simulink model "Proj2_INLC2"  (R2019b)
settings: Solver=VariableStepAuto  StartTime=0.0  StopTime=10.0  RelTol=1e-3
values from neighbouring files (symbols this model uses):
  a_phi_des = pi/2    (= 1.57079632679)    [project2_code.m]
  alpha_NL = 25    [project2_code.m]
  b_phi_des = [pi/2, pi/4]    [project2_code.m]
  beta_NL = 1    [project2_code.m]
  f_phi_des = 0.2    [project2_code.m]
  g = 9.8    [project2_code.m]
  Gamma_NL = eye(5)*1e-9    [project2_code.m]
  phi_des_bar = [pi/8, pi/4]    [project2_code.m]
  phi_dot_IC = [0; 0]    [project2_code.m]
  phi_dotdot_IC = [0; 0]    [project2_code.m]
  THD_IC = new_theta    [project2_code.m]
  theta = [theta1, theta2, theta3, theta4, theta5]    [project2_code.m]
settings Model: Creator=kaush  LastModifiedBy=kaush
settings DebuggingCC: SFMachineParentedDataDiag=error

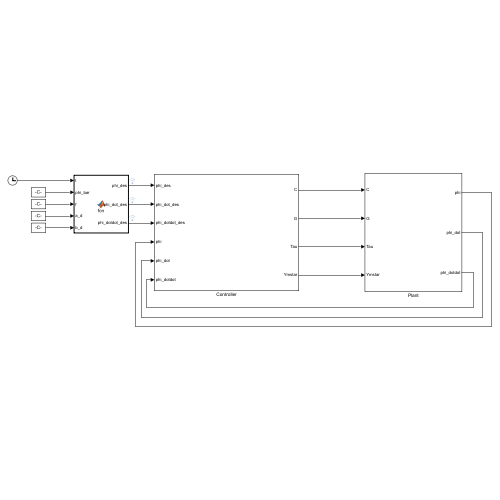
[thumbnail: Simulink's stored preview of the top-level diagram]
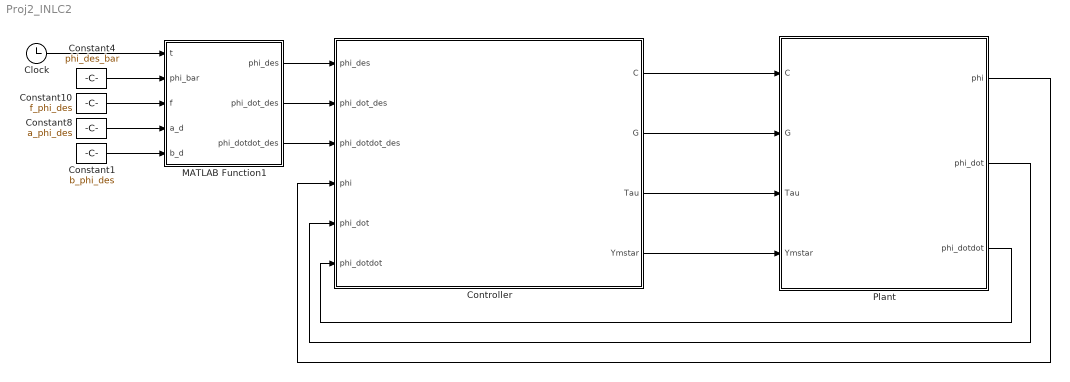
== system Proj2_INLC2 ==
  Clock : Clock
  Constant1 : Constant  Value=b_phi_des
  Constant10 : Constant  Value=f_phi_des
  Constant4 : Constant  Value=phi_des_bar
  Constant8 : Constant  Value=a_phi_des
  Controller : Subsystem
  MATLAB Function1 : MATLAB Function  TreatAsAtomicUnit=on
  Plant : Subsystem
  wires:
  Controller/1(C) -> Plant/1(C)
  Controller/3(Tau) -> Plant/3(Tau)
  Constant8/1 -> MATLAB Function1/4(a_d)
  Controller/2(G) -> Plant/2(G)
  MATLAB Function1/1(phi_des) -> Controller/1(phi_des)
  Clock/1 -> MATLAB Function1/1(t)
  MATLAB Function1/2(phi_dot_des) -> Controller/2(phi_dot_des)
  Plant/3(phi_dotdot) -> Controller/6(phi_dotdot)
  Plant/1(phi) -> Controller/4(phi)
  Constant4/1 -> MATLAB Function1/2(phi_bar)
  Plant/2(phi_dot) -> Controller/5(phi_dot)
  Constant1/1 -> MATLAB Function1/5(b_d)
  MATLAB Function1/3(phi_dotdot_des) -> Controller/3(phi_dotdot_des)
  Constant10/1 -> MATLAB Function1/3(f)
  Controller/4(Ymstar) -> Plant/4(Ymstar)

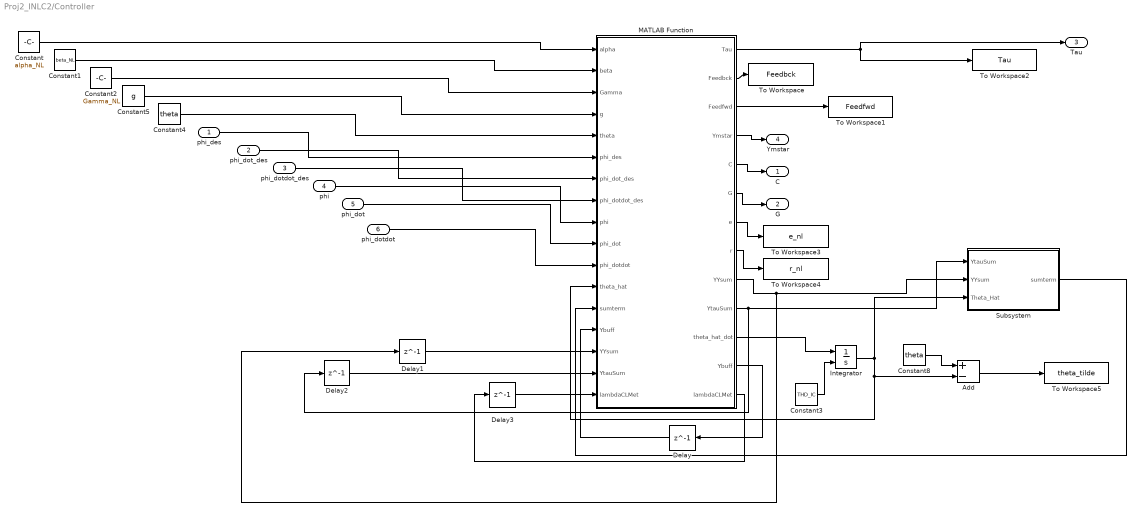
== system Proj2_INLC2/Controller ==
  phi_des : Inport
  phi_dot_des : Inport  Port=2
  phi_dotdot_des : Inport  Port=3
  phi : Inport  Port=4
  phi_dot : Inport  Port=5
  phi_dotdot : Inport  Port=6
  Add : Sum  Inputs=+-
  Constant : Constant  Value=alpha_NL
  Constant1 : Constant  Value=beta_NL
  Constant2 : Constant  Value=Gamma_NL
  Constant3 : Constant  Value=THD_IC
  Constant4 : Constant  Value=theta
  Constant5 : Constant  Value=g
  Constant8 : Constant  Value=theta
  Delay : Delay  DelayLength=1  InitialCondition=zeros(2,5,10)
  Delay1 : Delay  DelayLength=1  InitialCondition=zeros(5,5)
  Delay2 : Delay  DelayLength=1  InitialCondition=zeros(5,1)
  Delay3 : Delay  DelayLength=1  InitialCondition=0
  Integrator : Integrator  InitialConditionSource=external
  MATLAB Function : MATLAB Function  TreatAsAtomicUnit=on
  Subsystem : Subsystem
  To Workspace : ToWorkspace  VariableName=Feedbck  SaveFormat=Timeseries  SampleTime=-1
  To Workspace1 : ToWorkspace  VariableName=Feedfwd  SaveFormat=Timeseries  SampleTime=-1
  To Workspace2 : ToWorkspace  VariableName=Tau  SaveFormat=Timeseries  SampleTime=-1
  To Workspace3 : ToWorkspace  VariableName=e_nl  SaveFormat=Timeseries  SampleTime=-1
  To Workspace4 : ToWorkspace  VariableName=r_nl  SaveFormat=Timeseries  SampleTime=-1
  To Workspace5 : ToWorkspace  VariableName=theta_tilde  SaveFormat=Timeseries  SampleTime=-1
  C : Outport
  G : Outport  Port=2
  Tau : Outport  Port=3
  Ymstar : Outport  Port=4
  wires:
  phi_dotdot/1 -> MATLAB Function/11(phi_dotdot)
  phi_dot_des/1 -> MATLAB Function/7(phi_dot_des)
  phi/1 -> MATLAB Function/9(phi)
  MATLAB Function/11(theta_hat_dot) -> Integrator/1
  phi_dot/1 -> MATLAB Function/10(phi_dot)
  phi_des/1 -> MATLAB Function/6(phi_des)
  phi_dotdot_des/1 -> MATLAB Function/8(phi_dotdot_des)
  Constant/1 -> MATLAB Function/1(alpha)
  Constant1/1 -> MATLAB Function/2(beta)
  Constant2/1 -> MATLAB Function/3(Gamma)
  Constant3/1 -> Integrator/2
  Constant4/1 -> MATLAB Function/5(theta)
  MATLAB Function/5(C) -> C/1
  MATLAB Function/6(G) -> G/1
  MATLAB Function/1(Tau) -> Tau/1, To Workspace2/1
  MATLAB Function/2(Feedbck) -> To Workspace/1
  MATLAB Function/3(Feedfwd) -> To Workspace1/1
  Constant5/1 -> MATLAB Function/4(g)
  MATLAB Function/7(e) -> To Workspace3/1
  MATLAB Function/8(r) -> To Workspace4/1
  Constant8/1 -> Add/1
  Add/1 -> To Workspace5/1
  MATLAB Function/4(Ymstar) -> Ymstar/1
  Subsystem/1(sumterm) -> MATLAB Function/13(sumterm)
  MATLAB Function/9(YYsum) -> Subsystem/2(YYsum), Delay1/1
  Integrator/1 -> Subsystem/3(Theta_Hat), MATLAB Function/12(theta_hat), Add/2
  MATLAB Function/12(Ybuff) -> Delay/1
  Delay/1 -> MATLAB Function/14("Ybuff ")
  Delay1/1 -> MATLAB Function/15("YYsum ")
  Delay2/1 -> MATLAB Function/16("YtauSum ")
  MATLAB Function/10(YtauSum) -> Delay2/1, Subsystem/1(YtauSum)
  MATLAB Function/13(lambdaCLMet) -> Delay3/1
  Delay3/1 -> MATLAB Function/17("lambdaCLMet ")

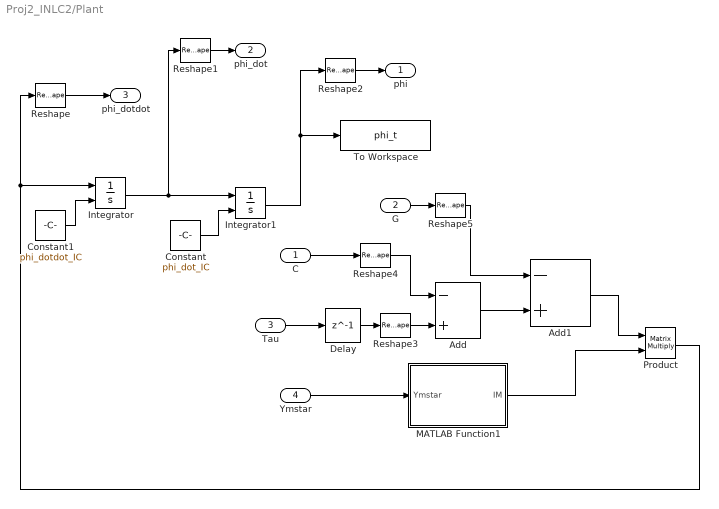
== system Proj2_INLC2/Plant ==
  C : Inport
  G : Inport  Port=2
  Tau : Inport  Port=3
  Ymstar : Inport  Port=4
  Add : Sum  Inputs=-+
  Add1 : Sum  Inputs=-+
  Constant : Constant  Value=phi_dot_IC
  Constant1 : Constant  Value=phi_dotdot_IC
  Delay : Delay  DelayLength=1
  Integrator : Integrator  InitialConditionSource=external
  Integrator1 : Integrator  InitialConditionSource=external
  MATLAB Function1 : MATLAB Function  TreatAsAtomicUnit=on
  Product : Product  Multiplication=Matrix(*)
  Reshape{,1..5} (6 alike) : Reshape
  To Workspace : ToWorkspace  VariableName=phi_t  SaveFormat=Timeseries  SampleTime=-1
  phi : Outport
  phi_dot : Outport  Port=2
  phi_dotdot : Outport  Port=3
  wires:
  Integrator/1 -> Reshape1/1, Integrator1/1
  Integrator1/1 -> To Workspace/1, Reshape2/1
  Constant1/1 -> Integrator/2
  Constant/1 -> Integrator1/2
  Tau/1 -> Delay/1
  Delay/1 -> Reshape3/1
  C/1 -> Reshape4/1
  G/1 -> Reshape5/1
  Product/1 -> Reshape/1, Integrator/1
  Ymstar/1 -> MATLAB Function1/1(Ymstar)
  Reshape/1 -> phi_dotdot/1
  Reshape1/1 -> phi_dot/1
  Reshape2/1 -> phi/1
  Add/1 -> Add1/2
  Add1/1 -> Product/1
  MATLAB Function1/1(IM) -> Product/2
  Reshape3/1 -> Add/2
  Reshape4/1 -> Add/1
  Reshape5/1 -> Add1/1

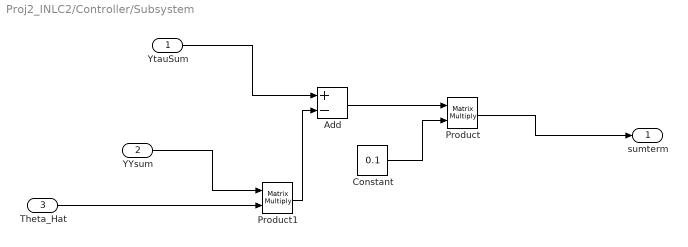
== system Proj2_INLC2/Controller/Subsystem ==
  YtauSum : Inport
  YYsum : Inport  Port=2  PortDimensions=[5,5]
  Theta_Hat : Inport  Port=3  PortDimensions=[5,1]
  Add : Sum  Inputs=+-
  Constant : Constant  Value=0.1
  Product : Product  Multiplication=Matrix(*)
  Product1 : Product  Multiplication=Matrix(*)
  sumterm : Outport
  wires:
  Constant/1 -> Product/2
  YYsum/1 -> Product1/1
  Add/1 -> Product/1
  Product/1 -> sumterm/1
  YtauSum/1 -> Add/1
  Theta_Hat/1 -> Product1/2
  Product1/1 -> Add/2

== matlab function Proj2_INLC2/Controller/MATLAB Function ==
  data: Tau output; Feedbck output; Feedfwd output; Ymstar output; C output; G output; e output; r output; YYsum output; YtauSum output; theta_hat_dot output; alpha input; beta input; Gamma input; g input; theta input; phi_des input; phi_dot_des input; phi_dotdot_des input; phi input; phi_dot input; phi_dotdot input; theta_hat input; sumterm input; Ybuff input; YYsum input; YtauSum input; Ybuff output; lambdaCLMet input; lambdaCLMet output
function [Tau, Feedbck, Feedfwd, Ymstar, C, G, e, r, YYsum, YtauSum, theta_hat_dot, Ybuff, lambdaCLMet] = fcn(alpha, beta, Gamma, g, theta, phi_des, phi_dot_des, phi_dotdot_des, phi, phi_dot, phi_dotdot, theta_hat, sumterm, Ybuff, YYsum, YtauSum, lambdaCLMet)
function [Tau, Feedbck, Feedfwd, Ymstar, C, G, e, r, YYsum, YtauSum, theta_hat_dot, Ybuff, lambdaCLMet] = fcn(alpha, beta, Gamma, g, theta, phi_des, phi_dot_des, phi_dotdot_des, phi, phi_dot, phi_dotdot, theta_hat, sumterm, Ybuff, YYsum, YtauSum, lambdaCLMet)
function [Tau, Feedbck, Feedfwd, Ymstar, C, G, e, r, YYsum, YtauSum, theta_hat_dot, Ybuff, lambdaCLMet] = fcn(alpha, beta, Gamma, g, theta, phi_des, phi_dot_des, phi_dotdot_des, phi, phi_dot, phi_dotdot, theta_hat, sumterm, Ybuff, YYsum, YtauSum, lambdaCLMet)

c1 = cos(phi(1));
c2 = cos(phi(2));
s1 = sin(phi(1));
s2 = sin(phi(2));
c12 = cos(phi(1) + phi(2));
s12 = sin(phi(1) + phi(2));

Ymstar = [theta(1) + 2*theta(2)*c2,theta(3)+theta(2)*c2; theta(3)+theta(2)*c2,theta(3)];
e = phi_des - phi;
e_dot = phi_dot_des - phi_dot;
% e_dotdot = phi_dotdot_des - phi_dotdot;
r = e_dot + alpha*e;
% r_dot = e_dotdot + alpha*e_dot;
eta = phi_dotdot_des + alpha*e_dot;
Y_M = [eta(1), (2*c2*eta(1)+ c2*eta(2)), eta(2), 0, 0; 0, (c2*eta(1)), (eta(1)+eta(2)), 0, 0];
M = Y_M*theta;
Y_C = [0, -(2*s2*phi_dot(1)*phi_dot(2)+s2*phi_dot(2)*phi_dot(2)), 0, 0, 0; 0, (s2*phi_dot(1)*phi_dot(1)), 0, 0, 0];
C = Y_C*theta;
Y_G = [0, 0, 0, (c1), (c12); 0, 0, 0, 0, (c12)];
G = Y_G*theta;
Y_MD = [0, -(2*s2*phi_dot(2)*r(1) + s2*phi_dot(2)*r(2)), 0, 0, 0; 0, (-s2*phi_dot(2)*r(1)), 0, 0, 0];
Y = Y_M + Y_C + Y_G + 0.5*Y_MD;
% theta_hat_dot = Gamma*(Y')*r;
Tau = Y*theta_hat + e + beta*r;
Feedbck = e + beta*r;
Feedfwd = Y*theta_hat;

% CL
% Ytau = Y'*Tau;
% YtYThetaHat = Y'*Y;

% Ybuff = zeros(2,5,100);
% YYsum = zeros(5,5);  YYsum, YtauSum, YYsumMinEig
% YtauSum = zeros(5,1);
YYsumMinEig = 0.0;
lambdaCL = 0.1;
% lambdaCLMet = false;
YYminDiff = 0.1;
if lambdaCLMet == 0
    YSV = svd(Y);
    if (min(YSV) > YYminDiff && norm(Tau) > YYminDiff)
        minDiff = 100.0;
        for Yi = 1:size(Ybuff,2)
                    YYdiffi = norm(Yi-Y);
                    if YYdiffi < minDiff
                        minDiff = YYdiffi;
                    end
        end            
        if minDiff > YYminDiff
                    Ybuff = circshift(Ybuff, 1); Ybuff(:,:,1) = Y;
                    YY = Y'*Y;
                    Ytau = Y'*Tau;
                    YYsum = YYsum + YY;
                    YtauSum = YtauSum + Ytau;
                    YYsumMinEig = min(eig(YYsum));
                    if YYsumMinEig > lambdaCL
%                         TCL = t
                        lambdaCLMet = 1;
                    end
        end
    end
end    

kcl = 0.1;
theta_hat_dot = Gamma*(Y')*r + Gamma*sumterm;

== matlab function Proj2_INLC2/MATLAB Function1 ==
  data: t input; phi_bar input; phi_des output; f input; a_d input; b_d input; phi_dot_des output; phi_dotdot_des output
% function [phi_des, phi_dot_des, phi_dotdot_des]= fcn(t,phi_des_bar, f_phi_des, a_phi_des, b_phi_des)
% phi_des = [phi_des_bar(1)*sin(2*pi*f_phi_des*t - a_phi_des)- b_phi_des(1); phi_des_bar(2)*sin(2*pi*f_phi_des*t - a_phi_des)+ b_phi_des(2)];
% phi_dot_des = [2*pi*f_phi_des*phi_des_bar(1)*cos(2*pi*f_phi_des*t - a_phi_des); 2*pi*f_phi_des*phi_des_bar(2)*cos(2*pi*f_phi_des*t - a_phi_des)];
% phi_dotdot_des = [-(2*pi*f_phi_des)*(2*pi*f_phi_des)*phi_des_bar(1)*sin(2*pi*f_phi_des*t - a_phi_des); -(2*pi*f_phi_des)*(2*pi*f_phi_des)*phi_des_bar(2)*sin(2*pi*f_phi_des*t - a_phi_des)];

function [phi_des, phi_dot_des, phi_dotdot_des]= fcn(t,phi_bar, f, a_d, b_d)
phi_des = [phi_bar(1)*sin(2*pi*f*t - a_d) - b_d(1); phi_bar(2)*sin(2*pi*f*t - a_d) + b_d(2)];
phi_dot_des = [2*pi*f*phi_bar(1)*cos(2*pi*f*t - a_d); 2*pi*f*phi_bar(2)*cos(2*pi*f*t - a_d)];
phi_dotdot_des = [-(2*pi*f)^(2)*phi_bar(1)*sin(2*pi*f*t - a_d); -(2*pi*f)^(2)*phi_bar(2)*sin(2*pi*f*t - a_d)];

== matlab function Proj2_INLC2/Plant/MATLAB Function1 ==
  data: Ymstar input; IM output
function IM = fcn( Ymstar)
IM = inv(Ymstar);
